simulink model "sampleModel1644"  (R2023a)
settings: Solver=VariableStepAuto  StartTime=0.0  StopTime=10.0  RelTol=1e-3
libraries: hdlsllib x6, simulink x3
settings Model: Creator=user1  LastModifiedBy=user1

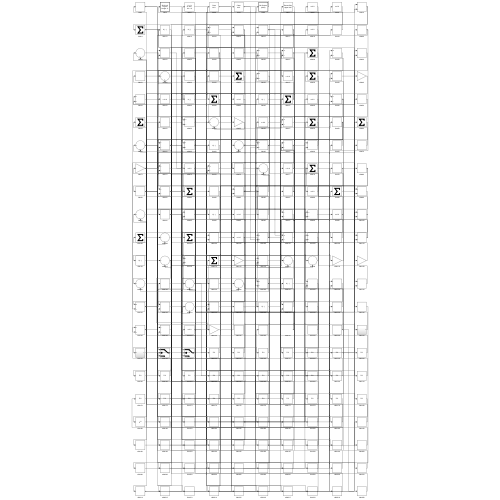
[thumbnail: Simulink's stored preview of the top-level diagram]
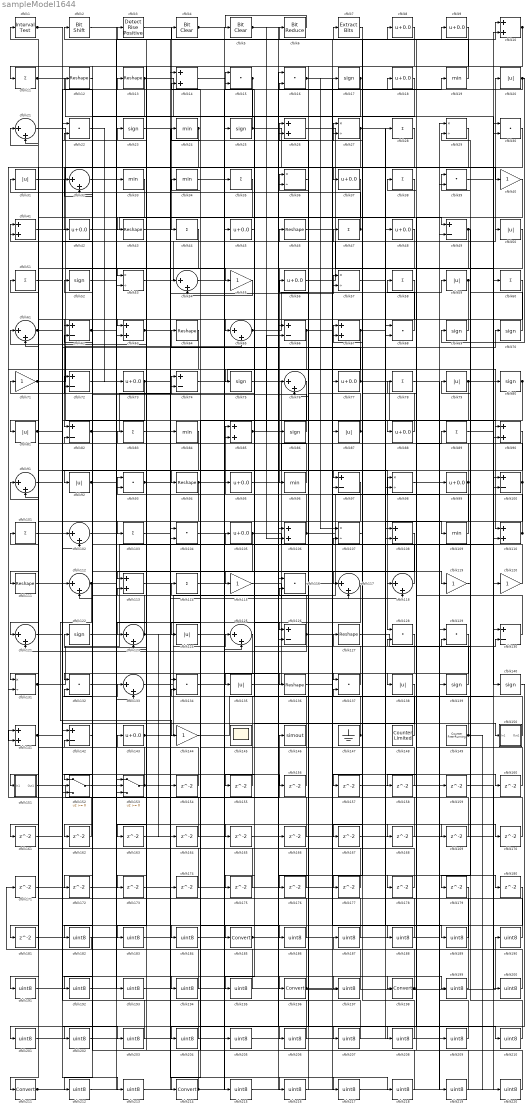
== system sampleModel1644 ==
  cfblk1 : hdlsllib/Logic and Bit Operations/Interval Test  IntervalClosedRight=on  uplimit=0.5  IntervalClosedLeft=on  lowlimit=-0.5  OutDataTypeStr=boolean
  cfblk{10,14,26,41,63,67,85,90,106,108,110,113,141} (13 alike) : Sum
  cfblk{49,62,66,72,74,82,97,100,126,130,142} (11 alike) : Sum  Inputs=+-
  cfblk{11,28,35,38,44,47,51,58,60,78,83,89,101,103,114} (15 alike) : Sum  Inputs=+
  cfblk{21,32,54,61,65,76,91,102,112,117..118,121,123,125,133} (15 alike) : Sum  Inputs=|++
  cfblk{15..16,22,30,39,68,93,104,116,128..129,132,134,137} (14 alike) : DotProduct  OutDataTypeStr=Inherit: Inherit via internal rule
  cfblk{8..9,18,37,42,45,48,56,73,77,88,95,99,105,143} (15 alike) : Bias  Bias=0.0  SaturateOnIntegerOverflow=off
  cfblk{27,29,36,53,57,98,107,131} (8 alike) : Product  Inputs=*/  RndMeth=Zero  SaturateOnIntegerOverflow=on
  cfblk{19,24,33..34,84,96,109} (7 alike) : MinMax
  cfblk{12..13,43,46,64,94,111,127,136} (9 alike) : Reshape
  cfblk{40,55,71,115,119..120,144} (7 alike) : Gain
  cfblk{17,23,25,52,69..70,75,80,86,122,139..140} (12 alike) : Signum
  cfblk{20,31,50,59,79,81,87,92,124,135,138} (11 alike) : Abs  SaturateOnIntegerOverflow=off
  cfblk145 : Scope
      settings: Floating=on
  cfblk146 : ToWorkspace  VariableName=simout  SaveFormat=Timeseries  SampleTime=-1
  cfblk147 : Ground
  cfblk148 : hdlsllib/Sources/Counter Limited  uplimit=7  tsamp=-1
  cfblk149 : hdlsllib/Sources/Counter Free-Running  NumBits=16  tsamp=-1
  cfblk150 : Subsystem
      settings: LibrarySourceBlock=|
      | hdlsllib/Ports &
      | Subsystems/Subsystem
  cfblk151 : Subsystem
      settings: LibrarySourceBlock=|
      | hdlsllib/Ports &
      | Subsystems/Subsystem
  cfblk152 : Switch  SaturateOnIntegerOverflow=off  InputSameDT=off
  cfblk153 : Switch  SaturateOnIntegerOverflow=off  InputSameDT=off
  cfblk{154..181} (28 alike) : Delay  SampleTime=1
  cfblk{182..184,186..195,197,199..210,212..213,215..220} (34 alike) : DataTypeConversion  OutDataTypeStr=uint8  SaturateOnIntegerOverflow=off  RndMeth=Floor
  cfblk{185,196,198,211,214} (5 alike) : DataTypeConversion  SaturateOnIntegerOverflow=off  RndMeth=Floor
  cfblk2 : hdlsllib/Logic and Bit Operations/Bit Shift  mode=Shift Left Logical  N=0
  cfblk3 : hdlsllib/Logic and Bit Operations/Detect Rise Positive  vinit=0  OutDataTypeStr=boolean
  cfblk4 : simulink/Logic and Bit Operations/Bit Clear  iBit=0
      settings: LibrarySourceBlock=|
      | hdlsllib/Logic and Bit
      | Operations/Bit Clear
  cfblk5 : simulink/Logic and Bit Operations/Bit Clear  iBit=0
      settings: LibrarySourceBlock=|
      | hdlsllib/Logic and Bit
      | Operations/Bit Clear
  cfblk6 : hdlsllib/Logic and Bit Operations/Bit Reduce  mode=AND
  cfblk7 : simulink/Logic and Bit Operations/Extract Bits  bitsToExtract=Upper half  numBits=8  bitIdxRange=[0 7]  outScalingMode=Preserve fixed-point scaling
      settings: LibrarySourceBlock=|
      | hdlsllib/Logic and Bit
      | Operations/Extract Bits
  wires:
  cfblk41/1 -> cfblk88/1
  cfblk22/1 -> cfblk73/1
  cfblk59/1 -> cfblk63/1, cfblk121/1, cfblk195/1
  cfblk30/1 -> cfblk211/1
  cfblk139/1 -> cfblk93/1
  cfblk149/1 -> cfblk122/1, cfblk220/1
  cfblk51/1 -> cfblk196/1
  cfblk135/1 -> cfblk89/1
  cfblk58/1 -> cfblk82/1
  cfblk120/1 -> cfblk41/1
  cfblk99/1 -> cfblk8/1, cfblk181/1
  cfblk8/1 -> cfblk103/1
  cfblk25/1 -> cfblk15/1, cfblk37/1
  cfblk1/1 -> cfblk184/1, cfblk203/1
  cfblk75/1 -> cfblk97/1
  cfblk143/1 -> cfblk125/1, cfblk164/1
  cfblk21/1 -> cfblk55/1
  cfblk74/1 -> cfblk110/1
  cfblk6/1 -> cfblk5/1
  cfblk3/1 -> cfblk44/1
  cfblk82/1 -> cfblk74/1, cfblk90/1
  cfblk29/1 -> cfblk42/1
  cfblk133/1 -> cfblk48/1
  cfblk53/1 -> cfblk20/1
  cfblk76/1 -> cfblk214/1
  cfblk46/1 -> cfblk97/2
  cfblk20/1 -> cfblk69/1, cfblk16/2
  cfblk50/1 -> cfblk137/1
  cfblk112/1 -> cfblk144/1, cfblk4/1
  cfblk79/1 -> cfblk130/1, cfblk126/2
  cfblk56/1 -> cfblk50/1
  cfblk131/1 -> cfblk100/1, cfblk47/1
  cfblk65/1 -> cfblk59/1, cfblk90/2
  cfblk113/1 -> cfblk57/1
  cfblk38/1 -> cfblk152/1
  cfblk10/1 -> cfblk132/1, cfblk11/1
  cfblk118/1 -> cfblk23/1
  cfblk73/1 -> cfblk10/1, cfblk152/3
  cfblk72/1 -> cfblk18/1
  cfblk67/1 -> cfblk28/1, cfblk141/2
  cfblk54/1 -> cfblk35/1
  cfblk40/1 -> cfblk138/1
  cfblk69/1 -> cfblk62/1
  cfblk19/1 -> cfblk2/1
  cfblk17/1 -> cfblk65/1, cfblk53/1
  cfblk45/1 -> cfblk135/1
  cfblk148/1 -> cfblk71/1
  cfblk37/1 -> cfblk151/1(In1)
  cfblk26/1 -> cfblk140/1
  cfblk152/1 -> cfblk33/1
  cfblk81/1 -> cfblk112/1, cfblk46/1, cfblk98/2
  cfblk106/1 -> cfblk3/1, cfblk36/1, cfblk39/2
  cfblk44/1 -> cfblk131/1
  cfblk68/1 -> cfblk58/1
  cfblk103/1 -> cfblk115/1
  cfblk92/1 -> cfblk168/1, cfblk169/1
  cfblk49/1 -> cfblk96/1, cfblk179/1
  cfblk109/1 -> cfblk67/1
  cfblk136/1 -> cfblk9/1
  cfblk39/1 -> cfblk120/1
  cfblk105/1 -> cfblk113/1, cfblk107/2
  cfblk31/1 -> cfblk40/1
  cfblk71/1 -> cfblk65/2, cfblk70/1
  cfblk80/1 -> cfblk124/1, cfblk158/1
  cfblk130/1 -> cfblk105/1
  cfblk137/1 -> cfblk72/1
  cfblk100/1 -> cfblk38/1, cfblk173/1
  cfblk91/1 -> cfblk185/1
  cfblk34/1 -> cfblk198/1
  cfblk86/1 -> cfblk22/2
  cfblk126/1 -> cfblk72/2, cfblk121/2, cfblk98/1
  cfblk63/1 -> cfblk165/1, cfblk207/1
  cfblk55/1 -> cfblk54/2
  cfblk57/1 -> cfblk109/1
  cfblk66/1 -> cfblk75/1, cfblk26/2, cfblk178/1
  cfblk110/1 -> cfblk85/1, cfblk14/2
  cfblk47/1 -> cfblk31/1, cfblk43/1
  cfblk101/1 -> cfblk150/1(In1)
  cfblk102/1 -> cfblk126/1
  cfblk11/1 -> cfblk153/1, cfblk100/2
  cfblk77/1 -> cfblk99/1, cfblk64/1
  cfblk64/1 -> cfblk81/1
  cfblk85/1 -> cfblk128/1, cfblk66/2, cfblk180/1
  cfblk27/1 -> cfblk111/1, cfblk189/1
  cfblk24/1 -> cfblk112/2, cfblk131/2
  cfblk61/1 -> cfblk102/2, cfblk213/1
  cfblk107/1 -> cfblk27/1
  cfblk144/1 -> cfblk80/1
  cfblk141/1 -> cfblk101/1, cfblk133/1
  cfblk2/1 -> cfblk94/1
  cfblk111/1 -> cfblk13/1
  cfblk124/1 -> cfblk19/1
  cfblk42/1 -> cfblk49/1
  cfblk4/1 -> cfblk95/1, cfblk136/1
  cfblk147/1 -> cfblk61/1, cfblk123/2
  cfblk5/1 -> cfblk86/1, cfblk106/2
  cfblk93/1 -> cfblk6/1, cfblk119/1
  cfblk87/1 -> cfblk56/1, cfblk167/1
  cfblk88/1 -> cfblk7/1
  cfblk70/1 -> cfblk39/1
  cfblk104/1 -> cfblk25/1
  cfblk119/1 -> cfblk79/1
  cfblk62/1 -> cfblk118/1, cfblk133/2
  cfblk15/1 -> cfblk123/1, cfblk53/2
  cfblk150/1(Out1) -> cfblk24/1
  cfblk153/1 -> cfblk52/1, cfblk197/1
  cfblk43/1 -> cfblk27/2
  cfblk96/1 -> cfblk21/2
  cfblk13/1 -> cfblk45/1, cfblk162/1
  cfblk95/1 -> cfblk106/1
  cfblk35/1 -> cfblk61/2
  cfblk90/1 -> cfblk92/1
  cfblk127/1 -> cfblk130/2
  cfblk151/1(Out1) -> cfblk146/1
  cfblk89/1 -> cfblk60/1
  cfblk18/1 -> cfblk117/1
  cfblk16/1 -> cfblk107/1, cfblk160/1
  cfblk115/1 -> cfblk118/2
  cfblk123/1 -> cfblk83/1, cfblk62/2, cfblk117/2, cfblk154/1, cfblk216/1
  cfblk9/1 -> cfblk66/1
  cfblk94/1 -> cfblk26/1, cfblk153/3
  cfblk154/1 -> cfblk1/1
  cfblk117/1 -> cfblk155/1
  cfblk155/1 -> cfblk22/1
  cfblk121/1 -> cfblk156/1
  cfblk156/1 -> cfblk15/2
  cfblk28/1 -> cfblk157/1
  cfblk157/1 -> cfblk110/2
  cfblk158/1 -> cfblk74/2
  cfblk160/1 -> cfblk128/2
  cfblk60/1 -> cfblk161/1
  cfblk161/1 -> cfblk102/1
  cfblk162/1 -> cfblk141/1
  cfblk125/1 -> cfblk163/1
  cfblk163/1 -> cfblk10/2
  cfblk164/1 -> cfblk153/2
  cfblk166/1 -> cfblk104/1
  cfblk167/1 -> cfblk49/2
  cfblk168/1 -> cfblk21/1
  cfblk169/1 -> cfblk67/2
  cfblk23/1 -> cfblk170/1
  cfblk170/1 -> cfblk29/2
  cfblk171/1 -> cfblk57/2
  cfblk12/1 -> cfblk172/1
  cfblk172/1 -> cfblk85/2
  cfblk173/1 -> cfblk54/1
  cfblk174/1 -> cfblk152/2
  cfblk138/1 -> cfblk175/1
  cfblk175/1 -> cfblk82/2
  cfblk36/1 -> cfblk176/1
  cfblk176/1 -> cfblk132/2
  cfblk7/1 -> cfblk177/1
  cfblk177/1 -> cfblk41/2
  cfblk178/1 -> cfblk113/2
  cfblk181/1 -> cfblk77/1
  cfblk108/1 -> cfblk182/1
  cfblk182/1 -> cfblk171/1
  cfblk48/1 -> cfblk183/1
  cfblk183/1 -> cfblk108/1
  cfblk184/1 -> cfblk108/2
  cfblk185/1 -> cfblk36/2, cfblk29/1
  cfblk132/1 -> cfblk186/1
  cfblk186/1 -> cfblk91/1
  cfblk179/1 -> cfblk187/1
  cfblk187/1 -> cfblk91/2
  cfblk116/1 -> cfblk188/1
  cfblk188/1 -> cfblk137/2
  cfblk189/1 -> cfblk116/1
  cfblk190/1 -> cfblk116/2
  cfblk84/1 -> cfblk191/1
  cfblk191/1 -> cfblk104/2
  cfblk128/1 -> cfblk192/1
  cfblk192/1 -> cfblk84/1
  cfblk32/1 -> cfblk193/1
  cfblk193/1 -> cfblk87/1
  cfblk122/1 -> cfblk194/1
  cfblk194/1 -> cfblk32/1
  cfblk195/1 -> cfblk32/2
  cfblk196/1 -> cfblk190/1, cfblk16/1
  cfblk197/1 -> cfblk51/1
  cfblk198/1 -> cfblk14/1, cfblk143/1
  cfblk52/1 -> cfblk199/1
  cfblk199/1 -> cfblk34/1
  cfblk159/1 -> cfblk200/1
  cfblk200/1 -> cfblk68/1
  cfblk140/1 -> cfblk201/1
  cfblk201/1 -> cfblk159/1
  cfblk142/1 -> cfblk202/1
  cfblk202/1 -> cfblk68/2
  cfblk203/1 -> cfblk142/1
  cfblk180/1 -> cfblk204/1
  cfblk204/1 -> cfblk142/2
  cfblk134/1 -> cfblk205/1
  cfblk205/1 -> cfblk166/1
  cfblk97/1 -> cfblk206/1
  cfblk206/1 -> cfblk134/1
  cfblk207/1 -> cfblk134/2
  cfblk129/1 -> cfblk208/1
  cfblk208/1 -> cfblk127/1
  cfblk98/1 -> cfblk209/1
  cfblk209/1 -> cfblk129/1
  cfblk165/1 -> cfblk210/1
  cfblk210/1 -> cfblk129/2
  cfblk211/1 -> cfblk174/1, cfblk63/2
  cfblk33/1 -> cfblk212/1
  cfblk212/1 -> cfblk30/1
  cfblk213/1 -> cfblk30/2
  cfblk214/1 -> cfblk12/1, cfblk17/1, cfblk125/2
  cfblk14/1 -> cfblk215/1
  cfblk215/1 -> cfblk76/1
  cfblk216/1 -> cfblk76/2
  cfblk114/1 -> cfblk217/1
  cfblk217/1 -> cfblk139/1
  cfblk83/1 -> cfblk218/1
  cfblk218/1 -> cfblk114/1
  cfblk78/1 -> cfblk219/1
  cfblk219/1 -> cfblk93/2
  cfblk220/1 -> cfblk78/1

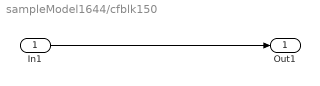
== system sampleModel1644/cfblk150 ==
  In1 : Inport
  Out1 : Outport
  wires:
  In1/1 -> Out1/1

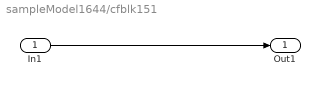
== system sampleModel1644/cfblk151 ==
  In1 : Inport
  Out1 : Outport
  wires:
  In1/1 -> Out1/1
